simulink model "LATC_Test_Calc2"  (R2021b)
settings: Solver=FixedStepDiscrete  StartTime=0.0  StopTime=inf  FixedStep=0.1  RelTol=1e-3
libraries: simulink x1
settings Model: DataDictionary=PubParsGlobal.sldd  Creator=GW00216231  LastModifiedBy=GW00216231
settings SolverCC: AlgebraicLoopSolver=TrustRegion
settings OptimizationCC: DefaultParameterBehavior=Inlined  EnhancedBackFolding=on  PassReuseOutputArgsThreshold=0  OptimizeBlockOrder=speed  DifferentSizesBufferReuse=on  OptimizationCustomize=off
settings DebuggingCC: SignalResolutionControl=TryResolveAllWithWarning  ParameterTunabilityLossMsg=error  SFMachineParentedDataDiag=warning  UnderSpecifiedDimensionMsg=warning
settings SFSimCC: MATLABDynamicMemAlloc=off
settings RTWCC: Description=Vector CANape/vSignalyzer Target (Visual C/C++ Project Makefile)  SystemTargetFile=cnp.tlc  TemplateMakefile=cnp_msdll.tmf
settings CodeAppCC: ForceParamTrailComments=on  OperatorAnnotations=on
settings STFCustomTargetCC: TargetLangStandard=C99 (ISO)  MATLABClassNameForMDSCustomization=Simulink.SoftwareTarget.TargetSpecificTriggerConfigurationBase  SystemTargetFile=cnp.tlc

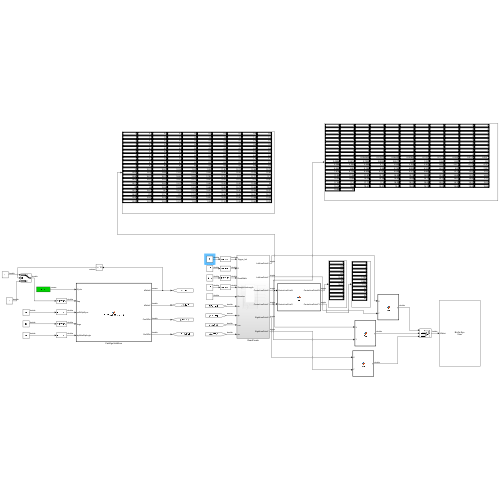
[thumbnail: Simulink's stored preview of the top-level diagram]
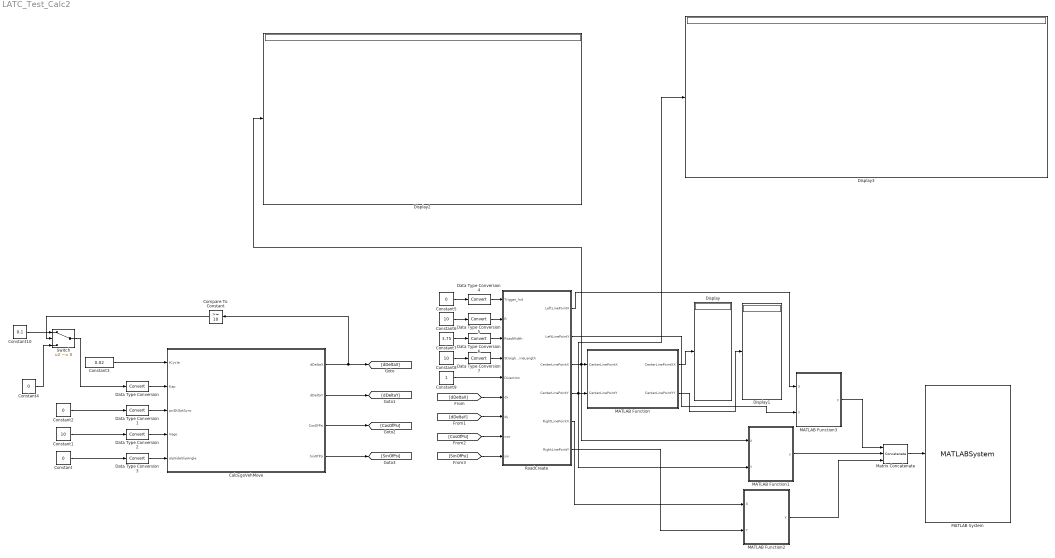
== system LATC_Test_Calc2 ==
  CalcEgoVehMove : MATLAB Function  TreatAsAtomicUnit=on
  Compare To Constant : simulink/Logic and Bit Operations/Compare To Constant  relop=>=  const=10  OutDataTypeStr=boolean
  Constant{,2,4..5} (4 alike) : Constant  Value=0
  Constant1 : Constant  Value=10
  Constant10 : Constant  Value=0.1
  Constant3 : Constant  Value=0.02
  Constant6 : Constant  Value=10
  Constant7 : Constant  Value=3.75
  Constant8 : Constant  Value=10
  Constant9 : Constant
  Data Type Conversion{,1..7} (8 alike) : DataTypeConversion
  Display{,1..3} (4 alike) : Display
  MATLAB Function : MATLAB Function  TreatAsAtomicUnit=on
  MATLAB Function1 : MATLAB Function  TreatAsAtomicUnit=on
  MATLAB Function2 : MATLAB Function  TreatAsAtomicUnit=on
  MATLAB Function3 : MATLAB Function  TreatAsAtomicUnit=on
  MATLAB System : MATLABSystem  System=BirdsEyeView17a  XLim=[ 0, 120 ]  YLim=[ -30, 30 ]  HasActors=off  ActorsColor=off  HasVision=on  HasRadar=off  HasRoads=off  HasLaneMarkings=off  Camera_Fov=52  Camera_Range=100  Camera_Yaw=0  Camera_Pos=[ 0, 0 ]  Radar_Fov=52  Radar_Range=100  Radar_Yaw=0  Radar_Pos=[ 0, 0 ]  MarkerSize=4  LabelFontSize=4  LabelOffset=[ 1.5, 1.5 ]  aspectratio=off
      mask Type: BirdsEyeView17a
      mask Display:
      | disp(['Bird''s-Eye' char(10) 'View']);
      | port_label('input',1,'Vision');
  Matrix Concatenate : Concatenate  NumInputs=3  Mode=Multidimensional array
  RoadCreate : Subsystem
  Switch : Switch  Criteria=u2 ~= 0
  wires:
  Constant8/1 -> Data Type Conversion7/1
  RoadCreate/3(CenterLinePointX) -> Display2/1, MATLAB Function/1(CenterLinePointX), MATLAB Function1/1(X)
  Constant2/1 -> Data Type Conversion1/1
  RoadCreate/4(CenterLinePointY) -> Display3/1, MATLAB Function1/2(Y), MATLAB Function/2(CenterLinePointY)
  Constant4/1 -> Switch/3
  Constant1/1 -> Data Type Conversion2/1
  Data Type Conversion2/1 -> CalcEgoVehMove/4(Vego)
  Data Type Conversion1/1 -> CalcEgoVehMove/3(psiDtOptSync)
  Constant9/1 -> RoadCreate/5(Direction)
  CalcEgoVehMove/1(dDeltaX) -> Compare To Constant/1, [dDeltaX]
  Constant6/1 -> Data Type Conversion5/1
  [SinOfPsi] -> RoadCreate/9(sin)
  Constant5/1 -> Data Type Conversion4/1
  Constant7/1 -> Data Type Conversion6/1
  [dDeltaX] -> RoadCreate/6(dx)
  Constant/1 -> Data Type Conversion3/1
  Constant3/1 -> CalcEgoVehMove/1(tCycle)
  CalcEgoVehMove/4(SinOfPsi) -> [SinOfPsi]
  Data Type Conversion3/1 -> CalcEgoVehMove/5(alpSideSlipAngle)
  [dDeltaY] -> RoadCreate/7(dy)
  CalcEgoVehMove/3(CosOfPsi) -> [CosOfPsi]
  Data Type Conversion/1 -> CalcEgoVehMove/2(Kap)
  [CosOfPsi] -> RoadCreate/8(cos)
  CalcEgoVehMove/2(dDeltaY) -> [dDeltaY]
  Data Type Conversion4/1 -> RoadCreate/1(Trigger_Init)
  Data Type Conversion5/1 -> RoadCreate/2(R)
  Data Type Conversion6/1 -> RoadCreate/3(RoadWidth)
  Data Type Conversion7/1 -> RoadCreate/4(StraightLineLength)
  MATLAB Function/1(CenterLinePointXX) -> Display/1
  MATLAB Function/2(CenterLinePointYY) -> Display1/1
  RoadCreate/5(RightLinePointX) -> MATLAB Function2/1(X)
  RoadCreate/6(RightLinePointY) -> MATLAB Function2/2(Y)
  RoadCreate/1(LeftLinePointX) -> MATLAB Function3/1(X)
  RoadCreate/2(LeftLinePointY) -> MATLAB Function3/2(Y)
  Matrix Concatenate/1 -> MATLAB System/1
  MATLAB Function3/1(y) -> Matrix Concatenate/1
  MATLAB Function1/1(y) -> Matrix Concatenate/2
  MATLAB Function2/1(y) -> Matrix Concatenate/3
  Compare To Constant/1 -> Switch/2
  Constant10/1 -> Switch/1
  Switch/1 -> Data Type Conversion/1

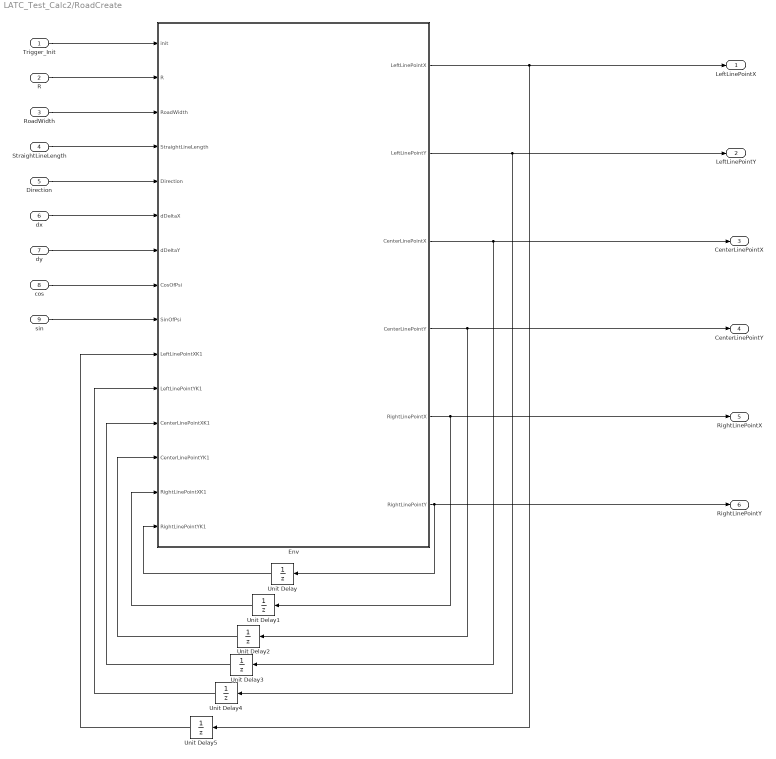
== system LATC_Test_Calc2/RoadCreate ==
  Trigger_Init : Inport
  R : Inport  Port=2
  RoadWidth : Inport  Port=3
  StraightLineLength : Inport  Port=4
  Direction : Inport  Port=5
  dx : Inport  Port=6
  dy : Inport  Port=7
  cos : Inport  Port=8
  sin : Inport  Port=9
  Env : MATLAB Function  TreatAsAtomicUnit=on
  Unit Delay{,1..5} (6 alike) : UnitDelay  SampleTime=-1  HasFrameUpgradeWarning=on
  LeftLinePointX : Outport
  LeftLinePointY : Outport  Port=2
  CenterLinePointX : Outport  Port=3
  CenterLinePointY : Outport  Port=4
  RightLinePointX : Outport  Port=5
  RightLinePointY : Outport  Port=6
  wires:
  Trigger_Init/1 -> Env/1(init)
  R/1 -> Env/2(R)
  RoadWidth/1 -> Env/3(RoadWidth)
  dx/1 -> Env/6(dDeltaX)
  cos/1 -> Env/8(CosOfPsi)
  dy/1 -> Env/7(dDeltaY)
  sin/1 -> Env/9(SinOfPsi)
  Env/6(RightLinePointY) -> RightLinePointY/1, Unit Delay/1
  Unit Delay/1 -> Env/15(RightLinePointYK1)
  Env/5(RightLinePointX) -> RightLinePointX/1, Unit Delay1/1
  Unit Delay1/1 -> Env/14(RightLinePointXK1)
  Env/4(CenterLinePointY) -> CenterLinePointY/1, Unit Delay2/1
  Unit Delay2/1 -> Env/13(CenterLinePointYK1)
  Env/3(CenterLinePointX) -> CenterLinePointX/1, Unit Delay3/1
  Unit Delay3/1 -> Env/12(CenterLinePointXK1)
  Env/2(LeftLinePointY) -> LeftLinePointY/1, Unit Delay4/1
  Unit Delay4/1 -> Env/11(LeftLinePointYK1)
  Env/1(LeftLinePointX) -> LeftLinePointX/1, Unit Delay5/1
  Unit Delay5/1 -> Env/10(LeftLinePointXK1)
  Direction/1 -> Env/5(Direction)
  StraightLineLength/1 -> Env/4(StraightLineLength)

== matlab function LATC_Test_Calc2/MATLAB Function2 ==
  data: X input; y output; Y input
function y = fcn(X,Y)

y = zeros(length(X),9);
for i = 1:1:length(X)
    y(i,1) = X(i);
    y(i,2) = Y(i);
    y(i,3) = 1;
    y(i,4) = 0;
    y(i,5) = 0;
    y(i,6) = i;
    y(i,7) = 0;
    y(i,8) = 1;
end
end

== matlab function LATC_Test_Calc2/MATLAB Function ==
  data: CenterLinePointX input; CenterLinePointXX output; CenterLinePointY input; CenterLinePointYY output
function [CenterLinePointXX,CenterLinePointYY]= fcn(CenterLinePointX,CenterLinePointY)
CenterLinePointXX = single(zeros(11,1));
CenterLinePointYY = single(zeros(11,1));
j = 1;
for i = 0:30:300
    if i==0
        i = 1;
    end
    CenterLinePointXX(j,1) = CenterLinePointX(i,1);
    CenterLinePointYY(j,1) = CenterLinePointY(i,1);
    j = j + 1;
end


end

== matlab function LATC_Test_Calc2/MATLAB Function3 ==
  data: X input; y output; Y input
function y = fcn(X,Y)

y = zeros(length(X),9);
for i = 1:1:length(X)
    y(i,1) = X(i);
    y(i,2) = Y(i);
    y(i,3) = 1;
    y(i,4) = 0;
    y(i,5) = 0;
    y(i,6) = i;
    y(i,7) = 0;
    y(i,8) = 1;
end
end

== matlab function LATC_Test_Calc2/RoadCreate/Env ==
  data: init input boolean; R input; RoadWidth input; StraightLineLength input; Direction input; dDeltaX input; dDeltaY input; CosOfPsi input; SinOfPsi input; LeftLinePointX output; LeftLinePointXK1 input single; LeftLinePointYK1 input single; CenterLinePointXK1 input single; CenterLinePointYK1 input single; LeftLinePointY output; RightLinePointXK1 input single; RightLinePointYK1 input single; CenterLinePointX output; CenterLinePointY output; RightLinePointX output; RightLinePointY output
function [LeftLinePointX,LeftLinePointY,CenterLinePointX,CenterLinePointY,RightLinePointX,RightLinePointY] = ...
    Env(init,R,RoadWidth,StraightLineLength,Direction,dDeltaX,dDeltaY,CosOfPsi,SinOfPsi,...
    LeftLinePointXK1,LeftLinePointYK1,CenterLinePointXK1,CenterLinePointYK1,RightLinePointXK1,RightLinePointYK1)

% R = single(20);                % m
% RoadWidth = single(3.75);       % m
% StraightLineLength =single(10); %m
% Direction = 1;

% R = R;                % m
% RoadWidth = RoadWidth;       % m
% StraightLineLength =single(10); %m
% Direction = 1;

LeftLinePointX = single(zeros(300,1));
LeftLinePointY = single(zeros(300,1));

CenterLinePointX = single(zeros(300,1));
CenterLinePointY = single(zeros(300,1));

RightLinePointX = single(zeros(300,1));
RightLinePointY = single(zeros(300,1));

LaneLeftPointX = single(zeros(100,1));
LaneLeftPointY = single(zeros(100,1));
LaneRightPointX = single(zeros(100,1));
LaneRightPointY = single(zeros(100,1));
LaneCenterPointX = single(zeros(100,1));
LaneCenterPointY = single(zeros(100,1));

StraightLaneLeft1_PointY = single(zeros(100,1));
StraightLaneLeft1_PointX = single(zeros(100,1));
StraightLaneRight1_PointY = single(zeros(100,1));
StraightLaneRight1_PointX = single(zeros(100,1));
StraightLaneCenter1_PointY = single(zeros(100,1));
StraightLaneCenter1_PointX = single(zeros(100,1));

StraightLaneLeft2_PointY = single(zeros(100,1));
StraightLaneLeft2_PointX = single(zeros(100,1));
StraightLaneRight2_PointY = single(zeros(100,1));
StraightLaneRight2_PointX = single(zeros(100,1));
StraightLaneCenter2_PointY = single(zeros(100,1));
StraightLaneCenter2_PointX = single(zeros(100,1));

if init==1
    if Direction == 1
        for i = 1:100
            LaneLeftPointX(i)=StraightLineLength+(R+RoadWidth/single(2))*sin((i-1)*pi/100);
            LaneLeftPointY(i)=R-(R+RoadWidth/single(2))*cos((i-1)*pi/100);
            LaneRightPointX(i)=StraightLineLength+(R-RoadWidth/single(2))*sin((i-1)*pi/100);
            LaneRightPointY(i)=R-(R-RoadWidth/single(2))*cos((i-1)*pi/100);

            LaneCenterPointX(i)=StraightLineLength+(R)*sin((i-1)*pi/100);
            LaneCenterPointY(i)=R-(R)*cos((i-1)*pi/100);
        end
        for i = 1:99
            StraightLaneLeft1_PointX(i+1) = i*(StraightLineLength/single(100));
            StraightLaneRight1_PointX(i+1) = i*(StraightLineLength/single(100));
            StraightLaneCenter1_PointX(i+1) = i*(StraightLineLength/single(100));

            StraightLaneLeft2_PointX(i+1) = i*(StraightLineLength/single(100));
            StraightLaneRight2_PointX(i+1) = i*(StraightLineLength/single(100));
            StraightLaneCenter2_PointX(i+1) = i*(StraightLineLength/single(100));
        end
        StraightLaneLeft2_PointX = StraightLaneLeft2_PointX(end:-1:1);
        StraightLaneRight2_PointX = StraightLaneRight2_PointX(end:-1:1);
        StraightLaneCenter2_PointX = StraightLaneCenter2_PointX(end:-1:1);

        for i = 1:100
            StraightLaneLeft1_PointY(i) = -(RoadWidth/single(2));
            StraightLaneRight1_PointY(i) = (RoadWidth/single(2));
            StraightLaneLeft2_PointY(i) = single(2)*R+(RoadWidth/single(2));
            StraightLaneRight2_PointY(i) = single(2)*R-(RoadWidth/single(2));
            StraightLaneCenter1_PointY(i) = single(0);
            StraightLaneCenter2_PointY(i) = single(2)*R;

        end

    else
        for i = 1:100
            LaneLeftPointX(i)=StraightLineLength+(R-RoadWidth/single(2))*sin((100-i)*pi/100);
            LaneLeftPointY(i)=-R-(R-RoadWidth/single(2))*cos((100-i)*pi/100);

            LaneRightPointX(i)=StraightLineLength+(R+RoadWidth/single(2))*sin((100-i)*pi/100);
            LaneRightPointY(i)=-R-(R+RoadWidth/single(2))*cos((100-i)*pi/100);

            LaneCenterPointX(i)=StraightLineLength+(R)*sin((100-i)*pi/100);
            LaneCenterPointY(i)=-R-(R)*cos((100-i)*pi/100);
        end
        for i = 1:99
            StraightLaneLeft1_PointX(i+1) = i*(StraightLineLength/single(100));
            StraightLaneRight1_PointX(i+1) = i*(StraightLineLength/single(100));
            StraightLaneCenter1_PointX(i+1) = i*(StraightLineLength/single(100));

            StraightLaneLeft2_PointX(i+1) = i*(StraightLineLength/single(100));
            StraightLaneRight2_PointX(i+1) = i*(StraightLineLength/single(100));
            StraightLaneCenter2_PointX(i+1) = i*(StraightLineLength/single(100));
        end
        StraightLaneLeft2_PointX = StraightLaneLeft2_PointX(end:-1:1);
        StraightLaneRight2_PointX = StraightLaneRight2_PointX(end:-1:1);
        StraightLaneCenter2_PointX = StraightLaneCenter2_PointX(end:-1:1);

        for i = 1:100
            StraightLaneLeft1_PointY(i) = -(RoadWidth/single(2));
            StraightLaneRight1_PointY(i) = (RoadWidth/single(2));

            StraightLaneLeft2_PointY(i) = -single(2)*R+(RoadWidth/single(2));
            StraightLaneRight2_PointY(i) = -single(2)*R-(RoadWidth/single(2));

            StraightLaneCenter1_PointY(i) = single(0);
            StraightLaneCenter2_PointY(i) = -single(2)*R;

        end

    end
    LeftLinePointX = [StraightLaneLeft1_PointX;LaneLeftPointX;StraightLaneLeft2_PointX];
    LeftLinePointY = [StraightLaneLeft1_PointY;LaneLeftPointY;StraightLaneLeft2_PointY];

    CenterLinePointX = [StraightLaneCenter1_PointX;LaneCenterPointX;StraightLaneCenter2_PointX];
    CenterLinePointY = [StraightLaneCenter1_PointY;LaneCenterPointY;StraightLaneCenter2_PointY];

    RightLinePointX = [StraightLaneRight1_PointX;LaneRightPointX;StraightLaneRight2_PointX];
    RightLinePointY = [StraightLaneRight1_PointY;LaneRightPointY;StraightLaneRight2_PointY]; 
else
    for i=1:300
        t_dx = LeftLinePointXK1(i)-dDeltaX;
        t_dy = LeftLinePointYK1(i)-dDeltaY;
        t_dxTmp = t_dx*CosOfPsi+t_dy*SinOfPsi;
        t_dyTmp = -t_dx*SinOfPsi+t_dy*CosOfPsi;
        LeftLinePointX(i) = t_dxTmp;
        LeftLinePointY(i) = t_dyTmp;

        ttt_dx = CenterLinePointXK1(i)-dDeltaX;
        ttt_dy = CenterLinePointYK1(i)-dDeltaY;
        ttt_dxTmp = ttt_dx*CosOfPsi+ttt_dy*SinOfPsi;
        ttt_dyTmp = -ttt_dx*SinOfPsi+ttt_dy*CosOfPsi;
        CenterLinePointX(i) = ttt_dxTmp;
        CenterLinePointY(i) = ttt_dyTmp;

        tt_dx = RightLinePointXK1(i)-dDeltaX;
        tt_dy = RightLinePointYK1(i)-dDeltaY;
        tt_dxTmp = tt_dx*CosOfPsi+tt_dy*SinOfPsi;
        tt_dyTmp = -tt_dx*SinOfPsi+tt_dy*CosOfPsi;
        RightLinePointX(i) = tt_dxTmp;
        RightLinePointY(i) = tt_dyTmp;
    end
end

== matlab function LATC_Test_Calc2/MATLAB Function1 ==
  data: X input; y output; Y input
function y = fcn(X,Y)

y = zeros(length(X),9);
for i = 1:1:length(X)
    y(i,1) = X(i);
    y(i,2) = Y(i);
    y(i,3) = 1;
    y(i,4) = 0;
    y(i,5) = 0;
    y(i,6) = i;
    y(i,7) = 0;
    y(i,8) = 1;
end
end

== matlab function LATC_Test_Calc2/CalcEgoVehMove ==
  data: dDeltaX output; tCycle input; Kap input; psiDtOptSync input; Vego input; alpSideSlipAngle input; dDeltaY output; CosOfPsi output; SinOfPsi output
function [dDeltaX,dDeltaY,CosOfPsi,SinOfPsi] = EgoVehicleMovement(tCycle,Kap,psiDtOptSync,Vego,alpSideSlipAngle)
%#codegen
if Kap==0
    dDeltaX = Vego*tCycle;
    dDeltaY = 0;
    CosOfPsi = 1;
    SinOfPsi = 0;
else
    t_kap = Kap;
    if ((Kap>0.125)||(Kap<-0.125))&&(Vego>1)
        t_kapPsiDtSync = psiDtOptSync/Vego;
        if abs(t_kapPsiDtSync)>abs(Kap)
            t_kap = t_kapPsiDtSync;
        end
    end
    t_Psi = t_kap*Vego*tCycle;
    SinOfPsi = sin(t_Psi);
    CosOfPsi = cos(t_Psi);
    t_dDeltaXTemp = SinOfPsi/t_kap;
    t_dDeltaYTemp = 2*(sin(t_Psi/2)*sin(t_Psi/2))/t_kap;
    dDeltaX = cos(alpSideSlipAngle)*t_dDeltaXTemp - sin(alpSideSlipAngle)*t_dDeltaYTemp;
    dDeltaY = sin(alpSideSlipAngle)*t_dDeltaXTemp + cos(alpSideSlipAngle)*t_dDeltaYTemp;
end
